simulink model "ThreePhasePDPWM"  (R2021b)
settings: Solver=ode45  StartTime=0.0  StopTime=0.5  MaxStep=1e-6  RelTol=1e-5
libraries: spsMosfetLib x24, simulink x12, spsDCVoltageSourceLib x6, spsVoltageMeasurementLib x3, spsGroundLib x2, spsThreePhaseSeriesRLCBranchLib x1, spspowerguiLib x1
settings Model: Creator=singh  LastModifiedBy=singh

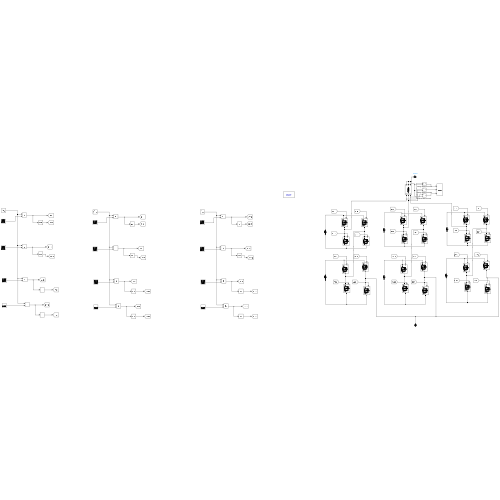
[thumbnail: Simulink's stored preview of the top-level diagram]
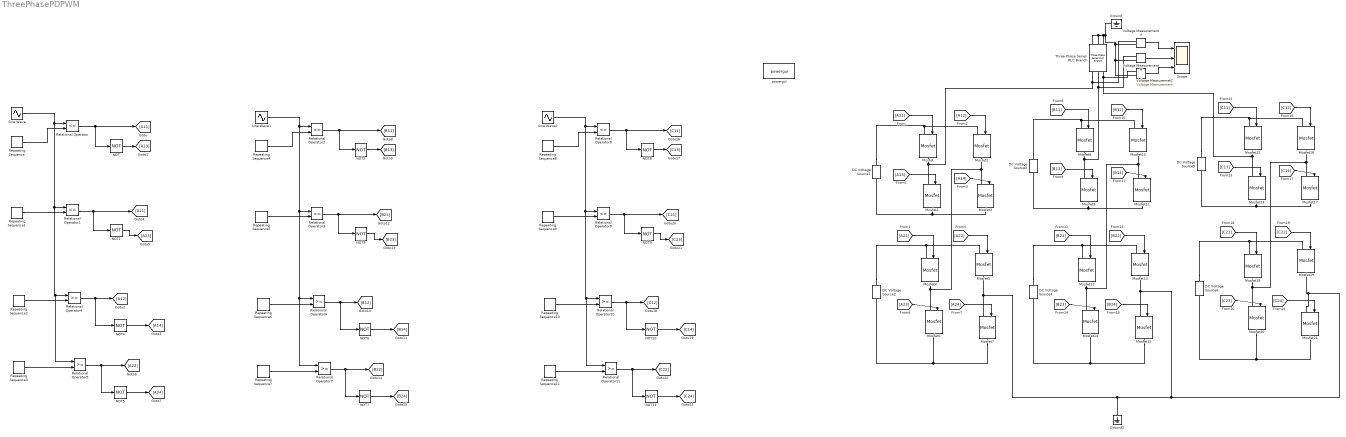
== system ThreePhasePDPWM ==
  DC Voltage Source{1..6} (6 alike) : spsDCVoltageSourceLib/DC Voltage Source  Amplitude=100  Measurements=None
  Ground : spsGroundLib/Ground  LConnTagsString=a
  Ground1 : spsGroundLib/Ground  LConnTagsString=a
  Mosfet{,1..23} (24 alike) : spsMosfetLib/Mosfet  Ron=0.1  Lon=0  Rd=0.01  Vfd=0  IC=0  Rs=1e5  Cs=inf  Measurements=off
  NOT{,1..11} (12 alike) : Logic  Operator=NOT  AllPortsSameDT=off  OutDataTypeStr=boolean
  Relational Operator{,1..3,8..9} (6 alike) : RelationalOperator  Operator=<=  OutDataTypeStr=boolean  RndMeth=Simplest
  Relational Operator{4..7,10..11} (6 alike) : RelationalOperator  OutDataTypeStr=boolean  RndMeth=Simplest
  Repeating Sequence : simulink/Sources/Repeating Sequence  rep_seq_t=[0 0.5 1]*1/10000  rep_seq_y=[0 1 0]
  Repeating Sequence1 : simulink/Sources/Repeating Sequence  rep_seq_t=[0 0.5 1]*1/10000  rep_seq_y=[1 2 1]
  Repeating Sequence10 : simulink/Sources/Repeating Sequence  rep_seq_t=[0 0.5 1]*1/10000  rep_seq_y=[-1 0 -1]
  Repeating Sequence11 : simulink/Sources/Repeating Sequence  rep_seq_t=[0 0.5 1]*1/10000  rep_seq_y=[-2 -1 -2]
  Repeating Sequence2 : simulink/Sources/Repeating Sequence  rep_seq_t=[0 0.5 1]*1/10000  rep_seq_y=[-1 0 -1]
  Repeating Sequence3 : simulink/Sources/Repeating Sequence  rep_seq_t=[0 0.5 1]*1/10000  rep_seq_y=[-2 -1 -2]
  Repeating Sequence4 : simulink/Sources/Repeating Sequence  rep_seq_t=[0 0.5 1]*1/10000  rep_seq_y=[0 1 0]
  Repeating Sequence5 : simulink/Sources/Repeating Sequence  rep_seq_t=[0 0.5 1]*1/10000  rep_seq_y=[1 2 1]
  Repeating Sequence6 : simulink/Sources/Repeating Sequence  rep_seq_t=[0 0.5 1]*1/10000  rep_seq_y=[-1 0 -1]
  Repeating Sequence7 : simulink/Sources/Repeating Sequence  rep_seq_t=[0 0.5 1]*1/10000  rep_seq_y=[-2 -1 -2]
  Repeating Sequence8 : simulink/Sources/Repeating Sequence  rep_seq_t=[0 0.5 1]*1/10000  rep_seq_y=[0 1 0]
  Repeating Sequence9 : simulink/Sources/Repeating Sequence  rep_seq_t=[0 0.5 1]*1/10000  rep_seq_y=[1 2 1]
  Scope : Scope  NumInputPorts=3
  Sine Wave : Sin  Amplitude=1.7  Frequency=50*2*pi  SampleTime=0
  Sine Wave1 : Sin  Amplitude=1.7  Frequency=50*2*pi  Phase=2*pi/3  SampleTime=0
  Sine Wave2 : Sin  Amplitude=1.7  Frequency=50*2*pi  Phase=4*pi/3  SampleTime=0
  Three-Phase Series RLC Branch : spsThreePhaseSeriesRLCBranchLib/Three-Phase Series RLC Branch  LConnTagsString=A|B|C  RConnTagsString=A|B|C  BranchType=R  Resistance=100  Inductance=1e-3  Capacitance=1e-6  Measurements=None
  Voltage MeasurementA : spsVoltageMeasurementLib/Voltage Measurement  PhasorSimulation=off  OutputType=Complex  PSBequivalent=0
  Voltage MeasurementB : spsVoltageMeasurementLib/Voltage Measurement  PhasorSimulation=off  OutputType=Complex  PSBequivalent=0
  Voltage MeasuremetC : spsVoltageMeasurementLib/Voltage Measurement  PhasorSimulation=off  OutputType=Complex  PSBequivalent=0
  powergui : spspowerguiLib/powergui  Priority=1  SimulationMode=Discrete  SampleTime=50e-6  frequency=60  Iterations=50  frequencyindice=0  Pbase=100e6  ErrMax=1e-4  UnitsV=kV  UnitsW=MW  buscounter=0  FunctionMessages=off  echomessages=off  EnableUseOfTLC=off  CurrentSourceSwitches=off  DisableSnubberDevices=off  DisableRonSwitches=off  DisableVfSwitches=off  DisplayEquations=off  AutomaticDiscreteSolvers=off  SolverType=Tustin/Backward Euler (TBE)  Interpol=off  ExternalGateDelay=off  methode=off  Ts=100  x0status=blocks  SPID=on  SwTol=0  HookPort=off  NonlinearTolerance=1e-4  nMaxIteration=100  ContinueOnMaxIteration=off  RestoreLinks=warning  ResistiveCurrentMeasurement=off  Frange=[0:2:500]  Ylog=off  Xlog=on  ShowGrid=off  save=off  variable=ZData  structure=0  ZoomFFT=off  StartTime=0.0  cycles=1  DisplayStyle=1  fundamental=60  FreqAxis=off  MaxFrequency=1000  frequencyindicesteady=1  RmsSteady=1  display=off
  wires:
  [A22] -> Mosfet5/1
  [A11] -> Mosfet/1
  [A12] -> Mosfet2/1
  [A13] -> Mosfet1/1
  [A24] -> Mosfet7/1
  [A21] -> Mosfet4/1
  [A23] -> Mosfet6/1
  [A14] -> Mosfet3/1
  [B22] -> Mosfet13/1
  [B11] -> Mosfet8/1
  [B12] -> Mosfet10/1
  [B13] -> Mosfet9/1
  [B24] -> Mosfet15/1
  [B21] -> Mosfet12/1
  [B23] -> Mosfet14/1
  [B14] -> Mosfet11/1
  [C14] -> Mosfet17/1
  [C23] -> Mosfet20/1
  [C13] -> Mosfet23/1
  [C21] -> Mosfet18/1
  [C24] -> Mosfet21/1
  [C12] -> Mosfet16/1
  [C11] -> Mosfet22/1
  [C22] -> Mosfet19/1
  NOT1/1 -> [A23]
  Sine Wave/1 -> Relational Operator5/1, Relational Operator4/1, Relational Operator1/1, Relational Operator/1
  Relational Operator4/1 -> [A12], NOT4/1
  NOT/1 -> [A13]
  Relational Operator5/1 -> [A22], NOT5/1
  Repeating Sequence1/1 -> Relational Operator1/2
  Repeating Sequence/1 -> Relational Operator/2
  NOT4/1 -> [A14]
  Repeating Sequence3/1 -> Relational Operator5/2
  NOT5/1 -> [A24]
  Repeating Sequence2/1 -> Relational Operator4/2
  Relational Operator1/1 -> NOT1/1, [A21]
  Relational Operator/1 -> NOT/1, [A11]
  Relational Operator2/1 -> NOT2/1, [B11]
  NOT7/1 -> [B24]
  Relational Operator3/1 -> NOT3/1, [B21]
  Repeating Sequence5/1 -> Relational Operator3/2
  Repeating Sequence4/1 -> Relational Operator2/2
  NOT6/1 -> [B14]
  Relational Operator7/1 -> [B22], NOT7/1
  Repeating Sequence7/1 -> Relational Operator7/2
  NOT2/1 -> [B13]
  Relational Operator6/1 -> [B12], NOT6/1
  Sine Wave1/1 -> Relational Operator7/1, Relational Operator6/1, Relational Operator3/1, Relational Operator2/1
  Repeating Sequence6/1 -> Relational Operator6/2
  NOT3/1 -> [B23]
  Relational Operator8/1 -> NOT8/1, [C11]
  NOT11/1 -> [C24]
  Relational Operator9/1 -> NOT9/1, [C21]
  Repeating Sequence9/1 -> Relational Operator9/2
  Repeating Sequence8/1 -> Relational Operator8/2
  NOT10/1 -> [C14]
  Relational Operator11/1 -> [C22], NOT11/1
  Repeating Sequence11/1 -> Relational Operator11/2
  NOT8/1 -> [C13]
  Relational Operator10/1 -> [C12], NOT10/1
  Sine Wave2/1 -> Relational Operator11/1, Relational Operator10/1, Relational Operator9/1, Relational Operator8/1
  Repeating Sequence10/1 -> Relational Operator10/2
  NOT9/1 -> [C23]
  Voltage MeasuremetC/1 -> Scope/3
  Voltage MeasurementB/1 -> Scope/2
  Voltage MeasurementA/1 -> Scope/1
  connections:
  DC Voltage Source2/RConn1 -- Mosfet4/LConn1 -- Mosfet5/LConn1
  Mosfet1/LConn1 -- Voltage MeasurementA/LConn1 -- Three-Phase Series RLC Branch/LConn1 -- Mosfet/RConn1
  DC Voltage Source1/RConn1 -- Mosfet/LConn1 -- Mosfet2/LConn1
  Mosfet3/LConn1 -- Mosfet6/LConn1 -- Mosfet4/RConn1 -- Mosfet2/RConn1
  DC Voltage Source1/LConn1 -- Mosfet1/RConn1 -- Mosfet3/RConn1
  Mosfet7/RConn1 -- Mosfet6/RConn1 -- DC Voltage Source2/LConn1
  DC Voltage Source4/RConn1 -- Mosfet12/LConn1 -- Mosfet13/LConn1
  Mosfet9/LConn1 -- Voltage MeasurementB/LConn1 -- Three-Phase Series RLC Branch/LConn2 -- Mosfet8/RConn1
  DC Voltage Source3/RConn1 -- Mosfet8/LConn1 -- Mosfet10/LConn1
  Mosfet11/LConn1 -- Mosfet14/LConn1 -- Mosfet12/RConn1 -- Mosfet10/RConn1
  DC Voltage Source3/LConn1 -- Mosfet9/RConn1 -- Mosfet11/RConn1
  Mosfet15/RConn1 -- Mosfet14/RConn1 -- DC Voltage Source4/LConn1
  Mosfet21/RConn1 -- Mosfet20/RConn1 -- DC Voltage Source6/LConn1
  DC Voltage Source6/RConn1 -- Mosfet18/LConn1 -- Mosfet19/LConn1
  DC Voltage Source5/RConn1 -- Mosfet22/LConn1 -- Mosfet16/LConn1
  DC Voltage Source5/LConn1 -- Mosfet23/RConn1 -- Mosfet17/RConn1
  Mosfet23/LConn1 -- Voltage MeasuremetC/LConn1 -- Three-Phase Series RLC Branch/LConn3 -- Mosfet22/RConn1
  Mosfet15/LConn1 -- Mosfet5/RConn1 -- Mosfet7/LConn1 -- Ground1/LConn1 -- Mosfet21/LConn1 -- Mosfet19/RConn1 -- Mosfet13/RConn1
  Mosfet17/LConn1 -- Mosfet20/LConn1 -- Mosfet18/RConn1 -- Mosfet16/RConn1
  Three-Phase Series RLC Branch/RConn1 -- Voltage MeasurementA/LConn2 -- Voltage MeasurementB/LConn2 -- Voltage MeasuremetC/LConn2 -- Ground/LConn1 -- Three-Phase Series RLC Branch/RConn3 -- Three-Phase Series RLC Branch/RConn2
